simulink model "accurateTiltingModel4"  (R2022b)
settings: Solver=ode4  StartTime=0.0  StopTime=10.0  FixedStep=0.001  RelTol=1e-3
undefined symbols (not defined in the file): alpha_0, beta, c_direction, I_b, I_i, k_m, k_t, m_b, N, p_mot, w_bar_0, x_0
libraries: uavutilslib x1
settings Model: Creator=pozzan  LastModifiedBy=pozzan

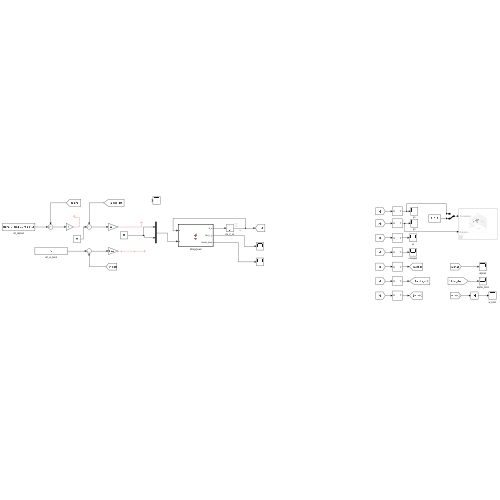
[thumbnail: Simulink's stored preview of the top-level diagram]
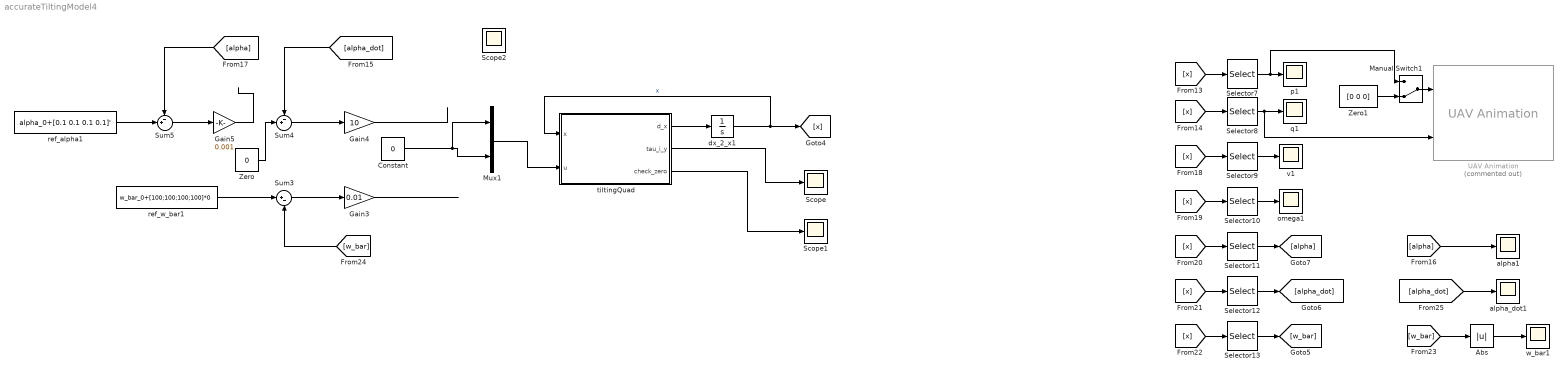
== system accurateTiltingModel4 ==
  Abs : Abs  SaturateOnIntegerOverflow=off
  Constant : Constant  Value=0
  Gain3 : Gain  Gain=0.01
  Gain4 : Gain  Gain=10
  Gain5 : Gain  Gain=0.001
  Manual Switch1 : ManualSwitch  CurrentSetting=0
  Mux1 : Mux  Inputs=2
  Scope : Scope
  Scope1 : Scope
  Scope2 : Scope
  Selector10 : Selector  InputPortWidth=13+3*N  IndexOptions=Index vector (dialog)  Indices=11:13  OutputSizes=1
  Selector11 : Selector  InputPortWidth=13+3*N  IndexOptions=Index vector (dialog)  Indices=14:14+N-1  OutputSizes=1
  Selector12 : Selector  InputPortWidth=13+3*N  IndexOptions=Index vector (dialog)  Indices=14+N:14+2*N-1  OutputSizes=1
  Selector13 : Selector  InputPortWidth=13+3*N  IndexOptions=Index vector (dialog)  Indices=14+2*N:14+3*N-1  OutputSizes=1
  Selector7 : Selector  InputPortWidth=13+3*N  IndexOptions=Index vector (dialog)  Indices=1:3  OutputSizes=1
  Selector8 : Selector  InputPortWidth=13+3*N  IndexOptions=Index vector (dialog)  Indices=4:7  OutputSizes=1
  Selector9 : Selector  InputPortWidth=13+3*N  IndexOptions=Index vector (dialog)  Indices=8:10  OutputSizes=1
  Sum3 : Sum  Inputs=|+-
  Sum4 : Sum  Inputs=-+|
  Sum5 : Sum  Inputs=-+|
  UAV Animation : uavutilslib/UAV Animation  Commented=on  UAVType=Multirotor  UAVSize=1  InertialZDirection=Up  SampleTime=0.02
  Zero : Constant  Value=0  OutDataTypeStr=Inherit: Inherit via back propagation
  Zero1 : Constant  Value=[0 0 0]  OutDataTypeStr=Inherit: Inherit via back propagation
  alpha1 : Scope
  alpha_dot1 : Scope
  dx_2_x1 : Integrator  InitialCondition=x_0
  omega1 : Scope
  p1 : Scope
  q1 : Scope
  ref_alpha1 : Constant  Value=alpha_0+[0.1 0.1 0.1 0.1]'  VectorParams1D=off
  ref_w_bar1 : Constant  Value=w_bar_0+[100;100;100;100]*0
  tiltingQuad : MATLAB Function  TreatAsAtomicUnit=on
  v1 : Scope
  w_bar1 : Scope
  wires:
  [w_bar] -> Abs/1
  Manual Switch1/1 -> UAV Animation/1
  Selector11/1 -> [alpha]
  Selector9/1 -> v1/1
  ref_alpha1/1 -> Sum5/2
  [x] -> Selector13/1
  Constant/1 -> Mux1/1, Mux1/2
  [alpha] -> alpha1/1
  [x] -> Selector8/1
  [alpha] -> Sum5/1
  [x] -> Selector10/1
  [alpha_dot] -> Sum4/1
  Sum5/1 -> Gain5/1
  Sum4/1 -> Gain4/1
  Gain3/1 -> ?
  dx_2_x1/1 -> [x], tiltingQuad/1(x)  "x"
  [x] -> Selector7/1
  Mux1/1 -> tiltingQuad/2(u)
  [alpha_dot] -> alpha_dot1/1
  Sum3/1 -> Gain3/1
  Selector13/1 -> [w_bar]
  [w_bar] -> Sum3/2
  Selector12/1 -> [alpha_dot]
  Zero1/1 -> Manual Switch1/2
  Selector7/1 -> Manual Switch1/1, p1/1
  Selector10/1 -> omega1/1
  Gain5/1 -> ?
  [x] -> Selector11/1
  [x] -> Selector12/1
  Abs/1 -> w_bar1/1
  tiltingQuad/1(d_x) -> dx_2_x1/1
  Selector8/1 -> UAV Animation/2, q1/1
  [x] -> Selector9/1
  ref_w_bar1/1 -> Sum3/1
  tiltingQuad/2(tau_i_y) -> Scope/1
  tiltingQuad/3(check_zero) -> Scope1/1
  Zero/1 -> Sum4/2
  Gain4/1 -> ?

== matlab function accurateTiltingModel4/tiltingQuad ==
  data: x input; u input; d_x output; m_b parameter; beta parameter; I_b parameter; I_i parameter; c_direction parameter; k_m parameter; k_t parameter; p_mot parameter; tau_i_y output; N parameter; check_zero output
function [d_x, tau_i_y, check_zero] = fcn(x, u, m_b, beta, I_b, I_i, c_direction, k_m, k_t, p_mot, N)

% state x: [p q v omega alpha alpha_dot w_bar]
% input u: [tau_i_x tau_i_z]
% output:
%   dot_x
%   tau_i_y: contraint torques
%   check_zero
% parameters
%   m_b: drone mass [kg]
%   beta: propellers tilting plane yaw angle [rad]
%   I_b: main body inertia [Kg*m^2]
%   I_i: rotor+propeller inertia [Kg*m^2]
%   c_direction: propeller tourning direction (1:CCW, -1:CW)
%   k_m: propeller drag coefficient [Nm/s^2]
%   k_t: propeller torque coefficient [Nm/s^2]
%   p_mot: rotor position w.r.t. body

p_ind = 1:3;
q_ind = 4:7;
v_ind = 8:10;
omega_ind = 11:13;
alpha_ind = 14:14+N-1;
alpha_dot_ind = 14+N:14+2*N-1;
w_bar_ind = 14+2*N:14+3*N-1;

tau_i_x_ind = 1:N;
tau_i_z_ind = N+1:2*N;



% position of c.o.m. w.r.t. globa frame
p = x(p_ind);
% quaternion associated to B2W rotation
q = x(q_ind);
% linear velocity of c.o.m. expressed in world frame
v = x(v_ind);
% angular velocity expressed in body frame
omega = x(omega_ind);
% tilting angles
alpha = x(alpha_ind);
% tilting angle rates
alpha_dot = x(alpha_dot_ind);
% spinning rate
w_bar = x(w_bar_ind);

% tilting angle accelerations
tau_i_x = u(tau_i_x_ind);
% spinning rate accelerations
tau_i_z = u(tau_i_z_ind);

% output vector initialization
d_x = zeros(size(x));
tau_i_y = zeros(1:N,1);
alpha_ddot = zeros(size(alpha));
w_bar_dot = zeros(size(w_bar));

% % propeller torques composition
% tau_i = [
%     tau_i_x.'
%     z.'
%     tau_i_z.'
%     ];

% body to world quaternion manipulation
eta = q(1);
epsilon = q(2:4);
epsilon_x = [
    0 -epsilon(3) epsilon(2)
    epsilon(3) 0 -epsilon(1)
    -epsilon(2) epsilon(1) 0
    ]; 
Rq = eye(3) + 2*eta*epsilon_x + 2*epsilon_x^2;          % rotation matrix, body to world
Mq = [eta, -epsilon'; epsilon, eta*eye(3)+epsilon_x];   % quaternion composition matrix
d_q = 1/2*Mq*[0;omega];                                 % quaternion derivative

coriol_b = cross(omega,I_b*omega);                      % coriolis componentes of the body

T_b = zeros(3,1);                                       % total body thrust
tau_b = zeros(3,1);                                     % total body torque (due to thrust)
b_tau_i = zeros(3,1);                                   % total propellers torque in body frame

%% constraint computation
% the constraint is in the form A_c*x_c+B_c=0
% x_c is the rotor y axis torque tau_i_y

k=1;

% rotor to body rotation matrix
B_R_i = axang2rotm([0 0 1 beta(k)])*axang2rotm([1 0 0 alpha(k)]);
% time derivative of rotor to body rotation matrix
B_R_i_dot = B_R_i * ...
    [
    0       0       0
    0       0       -alpha_dot(k)
    0 alpha_dot(k)  0
    ];
% angular velocity of the rotor in the rotor frame
omega_i = B_R_i.' * omega + [alpha_dot(k); 0; w_bar(k)];
% thrust of i-th prop in **body** frame
T_i = B_R_i* [0;0;c_direction(k)*k_t*w_bar(k)*abs(w_bar(k))];
% body torquw in body frame
tau_b = tau_b + cross(p_mot(k,:)',T_i);

% A_c = I(2,2) with I the final equivalent inertia matrix on the prop side
I = I_i\(eye(3)+I_i*B_R_i.'*inv(I_b)*B_R_i);
A_c = I(2,2);

c = I_i * B_R_i_dot*omega + cross(omega_i, I_i*omega_i);

c2 = c + I_i*B_R_i.'*(I_b\(tau_b-coriol_b));

% tau_e_i, rotor drag torque = -k_m * omega_i_z * abs(omega_i_z)
tau_ei = [0;0; -k_m*omega_i(3)*abs(omega_i(3))];

c3 = c2 - tau_ei;

B_c = I(2,[1 3])*[tau_i_x(k); tau_i_z(k)] - [0 1 0]*(I_i\c3);

tau_i_y(k) = A_c\(-B_c);

% propeller torques composition
tau_i = [
    tau_i_x.'
    tau_i_y.'
    tau_i_z.'
    ];

T_b = T_b + T_i;
b_tau_i = b_tau_i + B_R_i*tau_i(:,k);


% for k=1:N
%     % rotor to body rotation matrix
%     B_R_i = axang2rotm([0 0 1 beta(k)])*axang2rotm([1 0 0 alpha(k)]);
% 
%     % thrust of i-th prop in **body** frame
%     T_i = B_R_i* [0;0;c_direction(k)*k_t*w_bar(k)*abs(w_bar(k))];
%     % update total torque in body frame
%     tau_b = tau_b + cross(p_mot(k,:)',T_i);
%     % update total thrust in body frame
%     T_b = T_b + T_i;
%     % update propellers torque in body frame
%     b_tau_i = b_tau_i + B_R_i*tau_i(:,k);
% 
%     
% end

d_v = [0;0;-9.81] + 1/m_b*Rq*T_b;
d_omega = I_b\(tau_b-coriol_b-b_tau_i);

% for k=1:N
%     % rotor to body rotation matrix
%     B_R_i = axang2rotm([0 0 1 beta(k)])*axang2rotm([1 0 0 alpha(k)]);
%     % time derivative of rotor to body rotation matrix
%     B_R_i_dot = B_R_i * [0 0 0; 0 0 -alpha_dot(k); 0 alpha_dot(k) 0];
%     % angular rate of the i-th rotor in the i-th rotor frame
%     omega_i = B_R_i.' * omega + [alpha_dot(k); 0; w_bar(k)];
%     
%     % drag torque
%     tau_ei = [0;0; -k_m*omega_i(3)*abs(omega_i(3))];
%     
%     % [ddot_alpha_1; 0; dot_w_bar_i]
%     d_omega_rel = I_i\(tau_i(:,k)+tau_ei-cross(omega_i,I_i*omega_i)) - ...
%         B_R_i.'*d_omega - B_R_i_dot.'*omega;
% 
%     alpha_ddot(k) = d_omega_rel(1);
%     tau_i_y(k) = d_omega_rel(2);
%     w_bar_dot(k) = d_omega_rel(3);
% end

d_omega_rel = I*tau_i - I_i\c3;

alpha_ddot = d_omega_rel(1);
check_zero = d_omega_rel(2);
w_bar_dot = d_omega_rel(3);

%% output filling

d_x(p_ind) = v;
d_x(q_ind) = d_q;
d_x(v_ind) = d_v;
d_x(omega_ind) = d_omega;
d_x(alpha_ind) = alpha_dot;
d_x(alpha_dot_ind) = alpha_ddot;
d_x(w_bar_ind) = w_bar_dot;
